simulink model "Model"  (R2017b)
settings: Solver=VariableStepAuto  StartTime=0.0  StopTime=10.0  RelTol=1e-3
undefined symbols (not defined in the file): add
settings Model: Creator=aarrieta  LastModifiedBy=aarrieta

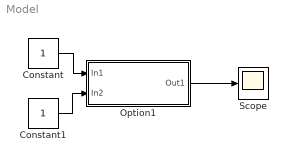
== system Model ==
  Constant : Constant
  Constant1 : Constant
  Option1 : Subsystem
  Scope : Scope
  wires:
  Constant/1 -> Option1/1(In1)
  Constant1/1 -> Option1/2(In2)
  Option1/1(Out1) -> Scope/1

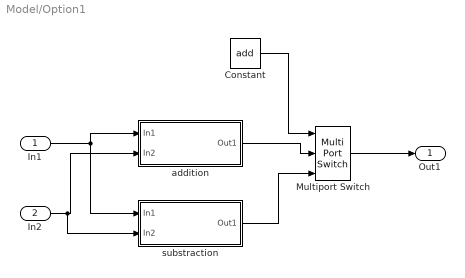
== system Model/Option1 ==
  In1 : Inport
  In2 : Inport  Port=2
  Constant : Constant  Value=add
  Multiport Switch : MultiPortSwitch  Inputs=2
  addition : Subsystem
  substraction : Subsystem
  Out1 : Outport
  wires:
  In1/1 -> substraction/1(In1), addition/1(In1)
  In2/1 -> substraction/2(In2), addition/2(In2)
  addition/1(Out1) -> Multiport Switch/2
  substraction/1(Out1) -> Multiport Switch/3
  Multiport Switch/1 -> Out1/1
  Constant/1 -> Multiport Switch/1

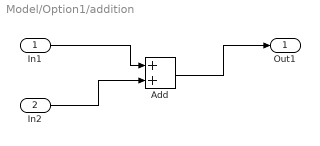
== system Model/Option1/addition ==
  In1 : Inport
  In2 : Inport  Port=2
  Add : Sum
  Out1 : Outport
  wires:
  In1/1 -> Add/1
  In2/1 -> Add/2
  Add/1 -> Out1/1

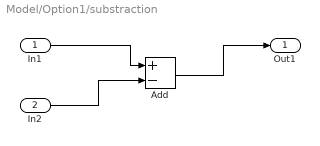
== system Model/Option1/substraction ==
  In1 : Inport
  In2 : Inport  Port=2
  Add : Sum  Inputs=+-
  Out1 : Outport
  wires:
  Add/1 -> Out1/1
  In2/1 -> Add/2
  In1/1 -> Add/1
